simulink subsystem "PieroModel"  (R2023b)
settings: Solver=VariableStepAuto  StartTime=0.0  StopTime=10.0  RelTol=1e-3
settings Model: Creator=chaya  LastModifiedBy=Usuario_UMA

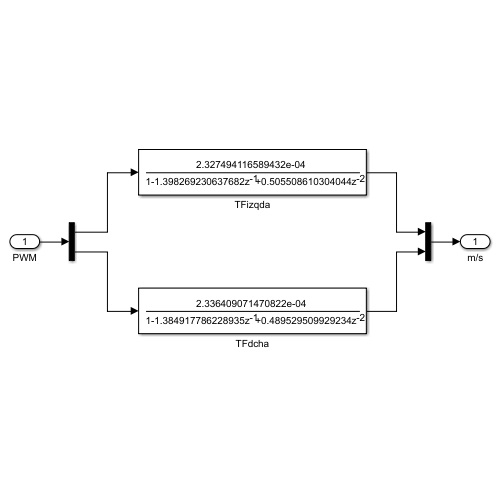
[thumbnail: Simulink's stored preview of the top-level diagram]
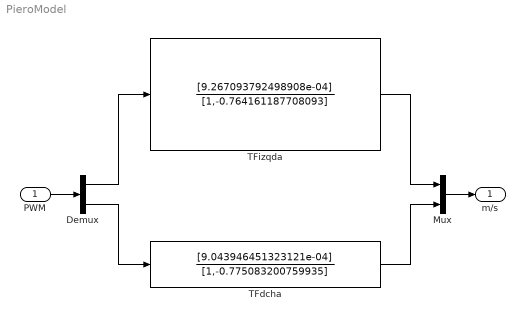
== system PieroModel ==
  PWM : Inport
  Demux : Demux  Outputs=2
  Mux : Mux  Inputs=2
  TFdcha : DiscreteFilter  Numerator=[9.043946451323121e-04]  Denominator=[1,-0.775083200759935]
  TFizqda : DiscreteFilter  Numerator=[9.267093792498908e-04]  Denominator=[1,-0.764161187708093]
  m/s : Outport
  wires:
  Mux/1 -> m/s/1
  PWM/1 -> Demux/1
  Demux/1 -> TFizqda/1
  TFizqda/1 -> Mux/1
  Demux/2 -> TFdcha/1
  TFdcha/1 -> Mux/2
